simulink model "zad8"  (R2016b)
settings: Solver=VariableStepAuto  StartTime=0.0  StopTime=10.0  RelTol=1e-3
values from neighbouring files (symbols this model uses):
  Ul = -1 : 0.01 : 1    [zad1_dod.m]    (also in zad6.m = -0.5)
undefined symbols (not defined in the file or in its folder): Tp
settings Model: Creator=tomasz  LastModifiedBy=tomasz

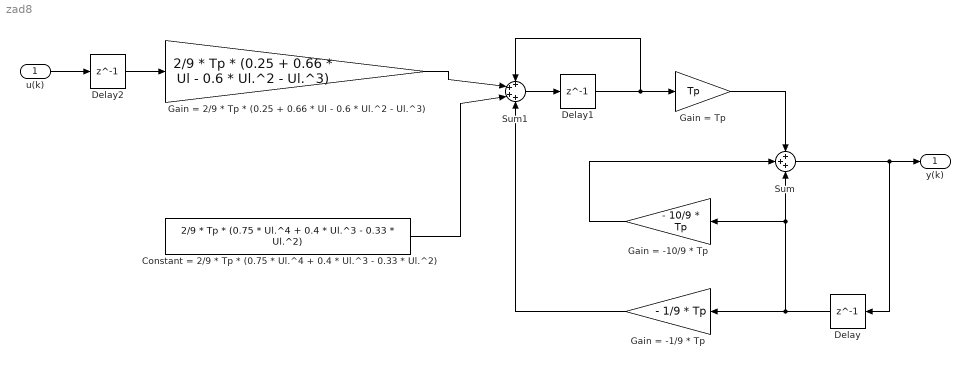
== system zad8 ==
  u(k) : Inport
  Constant = 2/9 * Tp * (0.75 * Ul.^4 + 0.4 * Ul.^3 - 0.33 * Ul.^2) : Constant  Value=2/9 * Tp * (0.75 * Ul.^4 + 0.4 * Ul.^3 - 0.33 * Ul.^2)
  Delay : Delay  DelayLength=1  InitialCondition=0
  Delay1 : Delay  DelayLength=1  InitialCondition=0
  Delay2 : Delay  DelayLength=1  InitialCondition=0
  Gain = -1/9 * Tp : Gain  Gain=- 1/9 * Tp
  Gain = -10/9 * Tp : Gain  Gain=- 10/9 * Tp
  Gain = 2/9 * Tp * (0.25 + 0.66 * Ul - 0.6 * Ul.^2 - Ul.^3) : Gain  Gain=2/9 * Tp * (0.25 + 0.66 * Ul - 0.6 * Ul.^2 - Ul.^3)
  Gain = Tp : Gain  Gain=Tp
  Sum : Sum  Inputs=+++
  Sum1 : Sum  Inputs=++++
  y(k) : Outport
  wires:
  Sum/1 -> Delay/1, y(k)/1
  Delay1/1 -> Sum1/1, Gain = Tp/1
  Delay/1 -> Gain = -1/9 * Tp/1, Gain = -10/9 * Tp/1, Sum/3
  Gain = -10/9 * Tp/1 -> Sum/2
  Gain = Tp/1 -> Sum/1
  Sum1/1 -> Delay1/1
  Gain = -1/9 * Tp/1 -> Sum1/4
  u(k)/1 -> Delay2/1
  Delay2/1 -> Gain = 2/9 * Tp * (0.25 + 0.66 * Ul - 0.6 * Ul.^2 - Ul.^3)/1
  Gain = 2/9 * Tp * (0.25 + 0.66 * Ul - 0.6 * Ul.^2 - Ul.^3)/1 -> Sum1/2
  Constant = 2/9 * Tp * (0.75 * Ul.^4 + 0.4 * Ul.^3 - 0.33 * Ul.^2)/1 -> Sum1/3
